simulink model "test_urarm_movejoints"  (R2014a)
settings: Solver=ode45  StartTime=0.0  StopTime=10.0  RelTol=1e-3
libraries: urarm_simulink x1
settings Model: Creator=fkzhang  LastModifiedBy=Marco
settings DataIOCC: SignalLoggingSaveFormat=ModelDataLogs
settings DebuggingCC: UnderspecifiedInitializationDetection=Classic  MultiTaskDSMMsg=warning  MultiTaskCondExecSysMsg=none  FcnCallInpInsideContextMsg=EnableAllAsWarning
settings RTWCC: IncludeERTFirstTime=on

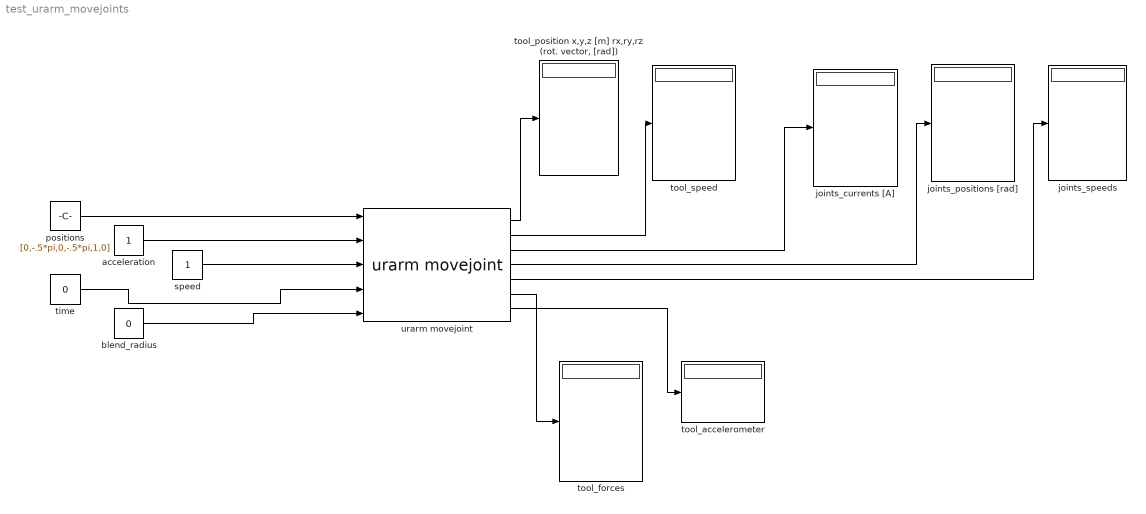
== system test_urarm_movejoints ==
  acceleration : Constant
  blend_radius : Constant  Value=0
  joints_currents [A] : Display
  joints_positions [rad] : Display
  joints_speeds : Display
  positions : Constant  Value=[0,-.5*pi,0,-.5*pi,1,0]
  speed : Constant
  time : Constant  Value=0
  tool_accelerometer : Display
  tool_forces : Display
  "tool_position x,y,z [m] rx,ry,rz (rot. vector, [rad])" : Display
  tool_speed : Display
  urarm movejoint : urarm_simulink/urarm movejoint  Ts=0
  wires:
  urarm movejoint/3 -> joints_currents [A]/1
  urarm movejoint/1 -> "tool_position x,y,z [m] rx,ry,rz (rot. vector, [rad])"/1
  urarm movejoint/2 -> tool_speed/1
  urarm movejoint/4 -> joints_positions [rad]/1
  urarm movejoint/5 -> joints_speeds/1
  urarm movejoint/6 -> tool_forces/1
  urarm movejoint/7 -> tool_accelerometer/1
  speed/1 -> urarm movejoint/3
  acceleration/1 -> urarm movejoint/2
  positions/1 -> urarm movejoint/1
  time/1 -> urarm movejoint/4
  blend_radius/1 -> urarm movejoint/5
